simulink model "mrsOmniwheelMPCModel"  (R2018b)
settings: Solver=VariableStepAuto  StartTime=0.0  StopTime=15  FixedStep=0.01  RelTol=1e-3  EnableMultiTasking=on
PreLoadFcn:
  | mrsOmniwheelMPCInit
undefined symbols (not defined in the file): sampleTime, waypoints
libraries: mobileRoboticsLib x3, mpclib x1
settings Model: EnablePacing=on  Creator=scastro  LastModifiedBy=scastro
settings DataIOCC: ExternalInput=[t,u]  LimitDataPoints=on
settings OptimizationCC: LifeSpan=inf
settings DebuggingCC: AllowSymbolicDim=off  LibraryContextMissingDiagnostic=none  SFUnexpectedBacktrackingDiag=warning  SFNoUnconditionalDefaultTransitionDiag=warning  SFExecutionAtInitializationDiag=none
settings SFSimCC: SimUseLocalCustomCode=off
settings RTWCC: RTWUseLocalCustomCode=off
settings CodeAppCC: StateflowObjectComments=on
settings GRTTargetCC: TargetLangStandard=C89/C90 (ANSI)  GeneratePreprocessorConditionals=Disable all
settings ConfigComp: CovMetricSettings=dw  CovHtmlReporting=on  CovSaveCumulativeToWorkspaceVar=on  CovSaveSingleToWorkspaceVar=on  CovExternalEMLEnable=off  CovSFcnEnable=off
settings SimscapeCC: SimscapeNominalValues="[{\"value\":\"10\",\"unit\":\"V\"},{\"value\":\"1\",\"unit\":\"A\"},{\"value\":\"10\",\"unit\":\"N*m\"},{\"value\":\"10\",\"unit\":\"bar\"},{\"value\":\"100\",\"unit\":\"kJ/kg\"},{\"value\":\"1\",\"unit\":\"kW\"},{\"value\":\"300\",\"unit\":\"K\"},{\"value\":\"100\",\"unit\":\"cm^3/s\"},{\"value\":\"1\",\"unit\":\"kN\"},{\"value\":\"1\",\"unit\":\"g/cm^3\"},{\"value\":\"1\",\"unit\":\"l\"},{\"value\":\"1\",\"unit\":\"cm^2\"},{\"value\":\"60\",\"unit\":\"Hz\"}]"  SimscapeLogType=all  SimscapeLogDataHistory=10000
settings ConfigurationSet: Description=SimMechanics 2G
settings ExplorerConfigSet: InternalSimMechanicsExplorerSettings="<ExplorerConfiguration><canonicalview>default</canonicalview><AnimationSetting><BasePlaybackSpeed>1.0</BasePlaybackSpeed><PlaybackSpeedFactor>1.0</PlaybackSpeedFactor></AnimationSetting><TilePanel><TileInfo><Tiles Columns=\"1\" Count=\"1\" Rows=\"1\"><Column Weight=\"1\"/><Row Weight=\"1\"/><Tile Height=\"1\" Width=\"1\" X=\"0\" Y=\"0\"/></Tiles></TileInfo><SceneInfo><SceneViewer><BGColor><R>0.60000002384185791</R><G>0.60000002384185791</G><B>0.60000002384185791</B></BGColor><Camera><DoPerspective>off</DoPerspective><Position><X>-1.70656042355848525</X><Y>-0.974920623359631922</Y><Z>4.72930454537082046</Z></Position><Center><X>0.552860638431633689</X><Y>1.42025063411503494</Y><Z>1.4843509506914252</Z></Center><Up><X>0.664249622453917166</X><Y>0.300615402055903091</Y><Z>0.684399604848363485</Z></Up><ViewLimDist>1</ViewLimDist><YLim>2.77881717169207398</YLim><XLim>3.55928742670435394</XLim></Camera></SceneViewer></SceneInfo></TilePanel><MechEditorPanel><Cameras/><GfxPanelCameraMap/><VideoCreator><PlaybackSpeedRatio>1.0</PlaybackSpeedRatio><FrameRate>30</FrameRate><VideoFormat>Motion JPEG AVI</VideoFormat><FrameSize>auto</FrameSize></VideoCreator></MechEditorPanel></ExplorerConfiguration>"

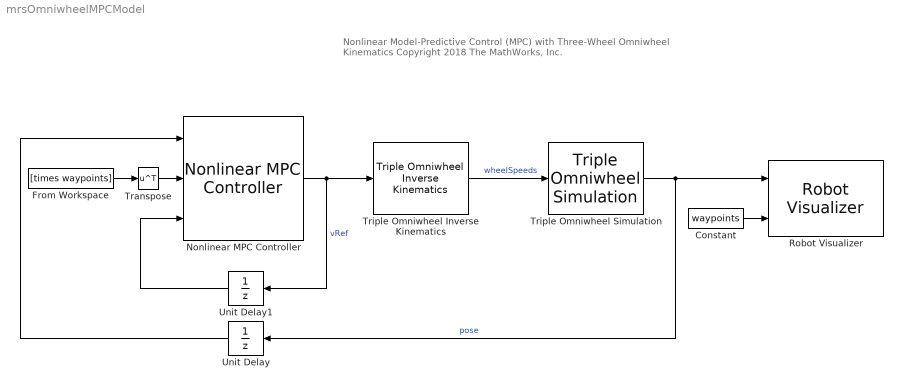
== system mrsOmniwheelMPCModel ==
  note: Nonlinear Model-Predictive Control (MPC)
      | with Three-Wheel Omniwheel Kinematics
      |
      | Copyright 2018 The MathWorks, Inc.
  Constant : Constant  Value=waypoints
  From Workspace : FromWorkspace  VariableName=[times waypoints]  SampleTime=sampleTime  OutputAfterFinalValue=Holding final value
  Nonlinear MPC Controller : mpclib/Nonlinear MPC Controller  SCDEnableBlockLinearizationSpecification=on  nlmpcobj=controller  UseObjectTs=on  md_enabled=off  param_enabled=off  cost_enabled=off  mvseq_enabled=off  stateseq_enabled=off  ovseq_enabled=off  slack_enabled=off  status_enabled=off  ov_min=off  ov_max=off  mv_min=off  mv_max=off  mvrate_min=off  mvrate_max=off  state_min=off  state_max=off  ov_weight=off  mv_weight=off  mvrate_weight=off  ecr_weight=off  mvtarget_enabled=off  nlp_initialize=off
      settings: SourceProductName=Model Predictive Control Toolbox
  Robot Visualizer : mobileRoboticsLib/Environments/Robot Visualizer  Priority=99  robotRadius=0  showTrajectory=on  hasWaypoints=on  hasLidar=off  sensorOffset=[ 0 0 ]  scanAngles=scanAngles  hasObjDetector=off  objDetectorOffset=[ 0, 0 ]  objDetectorAngle=0  objDetectorFOV=pi/4  objDetectorMaxRange=5  objectColors=[ 1, 0, 0; 0, 1, 0; 0, 0, 1 ]
  Transpose : Math  Operator=transpose  SaturateOnIntegerOverflow=on
  "Triple Omniwheel Inverse Kinematics " : mobileRoboticsLib/Kinematic Models/Triple Omniwheel/Triple Omniwheel Inverse Kinematics   wheelRadius=wheelRadius  robotRadius=robotRadius  wheelAngles=wheelAngles
      settings: SourceProductName=Mobile Robotics Simulation Toolbox
  Triple Omniwheel Simulation : mobileRoboticsLib/Kinematic Models/Triple Omniwheel/Triple Omniwheel Simulation  wheelRadius=wheelRadius  robotRadius=robotRadius  wheelAngles=wheelAngles  initX=0  initY=0  initAngle=0  Ts=sampleTime
      settings: SourceProductName=Mobile Robotics Simulation Toolbox
  Unit Delay : UnitDelay  SampleTime=sampleTime
  Unit Delay1 : UnitDelay  SampleTime=sampleTime
  wires:
  "Triple Omniwheel Inverse Kinematics "/1 -> Triple Omniwheel Simulation/1  "wheelSpeeds"
  Nonlinear MPC Controller/1 -> "Triple Omniwheel Inverse Kinematics "/1, Unit Delay1/1  "vRef"
  Triple Omniwheel Simulation/1 -> Robot Visualizer/1, Unit Delay/1  "pose"
  Unit Delay1/1 -> Nonlinear MPC Controller/3
  Unit Delay/1 -> Nonlinear MPC Controller/1
  Constant/1 -> Robot Visualizer/2
  From Workspace/1 -> Transpose/1
  Transpose/1 -> Nonlinear MPC Controller/2
